simulink model "mcb_pmsm_hall_offset_MCSPTE1AK144"  (R2021a)
settings: Solver=FixedStepDiscrete  StartTime=0.0  StopTime=10.0  FixedStep=0.001  RelTol=1e-3  EnableMultiTasking=on
PreLoadFcn:
  | mcb_pmsm_foc_hall_MCSPTE1AK144_data;
InitFcn:
  | mbd_s32k_consistency_checks(bdroot(gcs));
values from neighbouring files (symbols this model uses):
  PWM_frequency = 20e3    (= 20000)    [mcb_pmsm_foc_hall_MCSPTE1AK144_data.m]
  Ts = T_pwm * 2    (= 0.0001)    [mcb_pmsm_foc_hall_MCSPTE1AK144_data.m]
  Ts_uart = 0.01    [mcb_pmsm_foc_hall_MCSPTE1AK144_data.m]
undefined symbols (not defined in the file or in its folder): External, LQFP, One, pmsm, Shot, TRGMUX_PDB_TRIG
libraries: mbd_s32k1xx_ec_toolbox x34, simulink x9, mcbcontrolslib x5, hdlsllib x4, mbd_msd_ec_toolbox x4, mcbpositiondecoderlib x2
settings Model: Creator=nxf40284  LastModifiedBy=Prasad Hegde
settings SolverCC: AlgebraicLoopSolver=TrustRegion
settings DataIOCC: ExternalInput=off  InitialState=off  LimitDataPoints=on  SaveFormat=Array  SaveOutput=off  SignalLogging=off  SaveTime=off
settings OptimizationCC: DefaultParameterBehavior=Inlined  UseFloatMulNetSlope=on  DefaultUnderspecifiedDataType=single  UseSpecifiedMinMax=on  EnhancedBackFolding=on  PassReuseOutputArgsAs=Individual arguments  ZeroExternalMemoryAtStartup=off  ZeroInternalMemoryAtStartup=off  NoFixptDivByZeroProtection=on  EfficientFloat2IntCast=on  EfficientTunableParamExpr=on
settings DebuggingCC: MergeDetectMultiDrivingBlocksExec=none  InheritedTsInSrcMsg=none  MultiTaskDSMMsg=none  SingleTaskRateTransMsg=error  ParameterTunabilityLossMsg=error  UnconnectedInputMsg=error  UnconnectedOutputMsg=error  UnconnectedLineMsg=error  AllowSymbolicDim=off  UnknownTsInhSupMsg=error  SFMachineParentedDataDiag=warning  ArithmeticOperatorsInVariantConditions=warning
settings HardwareCC: ProdBitPerPointer=32  ProdBitPerSizeT=32  ProdBitPerPtrDiffT=32  ProdLargestAtomicInteger=Long  ProdLargestAtomicFloat=Double  ProdWordSize=32  ProdHWDeviceType=ARM Compatible->ARM Cortex
settings SFSimCC: MATLABDynamicMemAlloc=off
settings RTWCC: Description=Model Based Design Toolbox S32K1xx Code Generation Target  SystemTargetFile=mbd_s32k.tlc  MakeCommand=mbd_s32k_make_rtw COPY_MDLREF_INCLUDES=0  TemplateMakefile=mbd_s32k.tmf
settings CodeAppCC: ForceParamTrailComments=on  IgnoreCustomStorageClasses=off  OperatorAnnotations=on  SimulinkDataObjDesc=on  SFDataObjDesc=on  InsertBlockDesc=on  StateflowObjectComments=on
settings STFCustomTargetCC: MultiwordLength=256  CombineOutputUpdateFcns=on  ERTCustomFileBanners=on  SupportContinuousTime=off  SupportNonInlinedSFcns=off  MATLABClassNameForMDSCustomization=Simulink.SoftwareTarget.ERTCustomization  GRTInterface=off  UseToolchainInfoCompliant=off  SystemTargetFile=mbd_s32k.tlc
settings ERTTargetCC: ParMdlRefBuildCompliant=off  CompOptLevelCompliant=off  ConcurrentExecutionCompliant=off  RemoveResetFunc=off  ModelStepFunctionPrototypeControlCompliant=off  CPPClassGenCompliant=off  UseToolchainInfoCompliant=off  InlinedParameterPlacement=NonHierarchical  ERTSrcFileBannerTemplate=mbd_ert_code_template.cgt  ERTHdrFileBannerTemplate=mbd_ert_code_template.cgt  ERTDataSrcFileTemplate=mbd_ert_code_template.cgt  ERTDataHdrFileTemplate=mbd_ert_code_template.cgt  ERTCustomFileTemplate=example_file_process.tlc

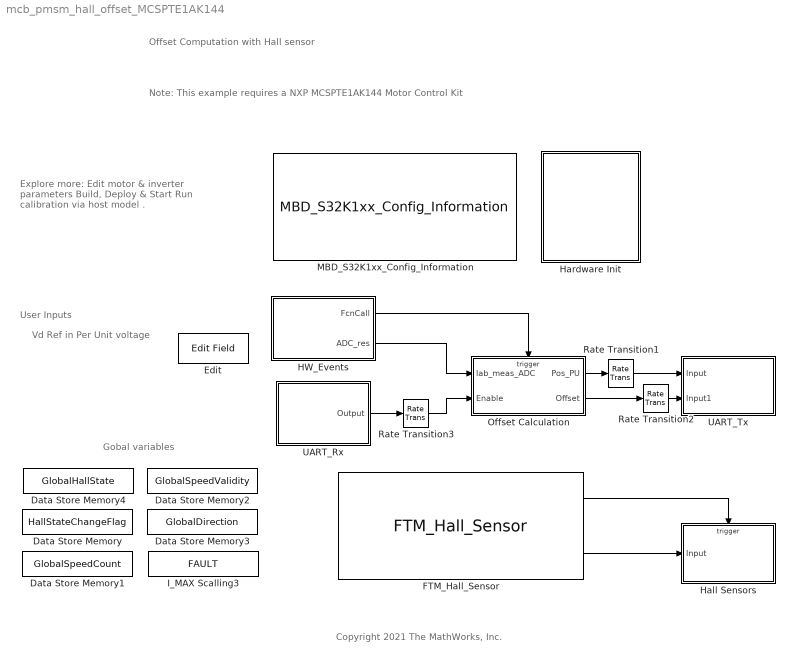
== system mcb_pmsm_hall_offset_MCSPTE1AK144 ==
  note: Note: This example requires a NXP MCSPTE1AK144 Motor Control Kit
  note: User Inputs
  note: Offset Computation with Hall sensor
  note: Vd Ref in Per Unit
      | voltage
  note: Gobal variables
  note: Copyright 2021 The MathWorks, Inc.
  note: Explore more:
      | Edit motor & inverter parameters
      | Build, Deploy & Start
      | Run calibration via host model .
  Data Store Memory : DataStoreMemory  DataStoreName=HallStateChangeFlag  ShowAdditionalParam=off
  Data Store Memory1 : DataStoreMemory  DataStoreName=GlobalSpeedCount  ShowAdditionalParam=off  OutDataTypeStr=uint16
  Data Store Memory2 : DataStoreMemory  DataStoreName=GlobalSpeedValidity  ShowAdditionalParam=off
  Data Store Memory3 : DataStoreMemory  DataStoreName=GlobalDirection  ShowAdditionalParam=off
  Data Store Memory4 : DataStoreMemory  DataStoreName=GlobalHallState  ShowAdditionalParam=off  OutDataTypeStr=uint32
  Edit : EditField  LabelPosition=Hide  ShowInitialText=on  Alignment=Center
  FTM_Hall_Sensor : mbd_s32k1xx_ec_toolbox/Motor Control Blocks/FTM Blocks/FTM_Hall_Sensor  e_mode=Rising or Falling  prescaler=128  max_period=0.10486  isrlevel=5  mcuTargetUpdate=on  filter_en=off  filter_value=0  pinFtm1Ch1=PTA1: [FTM1_CH1 | FTM Channel]  pinFtm2Ch0=PTD10: [FTM2_CH0 | FTM Channel]  pinFtm2Ch1=PTD11: [FTM2_CH1 | FTM Channel]
  HW_Events : Subsystem  TreatAsAtomicUnit=on
  Hall Sensors : Subsystem
  Hardware Init : Subsystem  Priority=2  TreatAsAtomicUnit=on
  I_MAX Scalling3 : DataStoreMemory  DataStoreName=FAULT  ReadBeforeWriteMsg=warning  WriteAfterWriteMsg=warning  WriteAfterReadMsg=warning  ShowAdditionalParam=off  OutDataTypeStr=boolean
  MBD_S32K1xx_Config_Information : mbd_s32k1xx_ec_toolbox/MBD_S32K1xx_Config_Information  Priority=1  mbdt_ver=0  disp_str=|  config_params=[]  mcu_target_name=S32K144  mcu_target_package=100-LQFP  mcu_target_sram_size=64KB  mcu_system_clock_freq=80  mcu_xtal_freq=External 8  mcu_steptick_timer=LPIT Channel 0  mcu_steptick_prio=10  ds_import_enable=on  target_compiler=GCC  target_memory=FLASH  gcc_target_compile_opts=-mcpu=cortex-m4 -mthumb -mfloat-abi=hard -mfpu=fpv4-sp-d16 -O1 -g -gstrict-dwarf  gcc_target_assemble_opts=-mcpu=cortex-m4 -mthumb -mfloat-abi=hard -mfpu=fpv4-sp-d16 -g  gcc_target_link_opts=-mcpu=cortex-m4 -mthumb -mfloat-abi=hard -mfpu=fpv4-sp-d16  gcc_target_default_lcf=on  gcc_target_user_lcf=S32K148_192_flash.ld  ghs_target_compile_opts=-cpu=cortexm4f -thumb -DARM_MATH_CM4 -fpu=vfpv4_d16 -fsingle -Ogeneral -Wundef -Wimplicit-int -Wshadow -Wtrigraphs --no_commons --gnu_asm -gnu99 -gdwarf-2 -G  ghs_target_assemble_opts=-cpu=cortexm4f -fpu=vfpv4_d16  ghs_target_link_opts=-cpu=cortexm4f -thumb -fpu=vfpv4_d16  ghs_target_default_lcf=on  ghs_target_user_lcf=S32K148_192_flash.ld  iar_target_compile_opts=--cpu=Cortex-M4F --thumb --fpu=VFPv4_sp -Ol -e --debug --dlib_config normal  iar_target_assemble_opts=--cpu Cortex-M4F --thumb --fpu VFPv4_sp  iar_target_link_opts=--no_exceptions --vfe --inline  iar_target_default_lcf=on  iar_target_user_lcf=S32K148_192_flash.icf  pil_download_enable=off  rbl_download_enable=on  rbl_start_delay=5000  rbl_download_interface=OpenSDA  rbl_restart_request=off  rbl_com_port=Custom  rbl_com_port_custom=COM1  pil_download_rate=57600  pil_opensda_drive=Custom  pil_opensda_drive_custom=D  pil_uart_instance=1  pil_uart_rx=PTC6: [LPUART1_RX | Receive]  pil_uart_tx=PTC7: [LPUART1_TX | Transmit]  FTM_PWM_PcrCheckEnDis=on  FTM_Input_Edge_Inputs_PcrCheckEnDis=on  FTM_Dual_Edge_Inputs_PcrCheckEnDis=on  FTM_Quadrature_Inputs_PcrCheckEnDis=on  FTM_Hall_Sensor_Inputs_PcrCheckEnDis=on  LPTMR_PcrCheckEnDis=on  PIT_PcrCheckEnDis=on  RTC_PcrCheckEnDis=on  FlexCAN_PcrCheckEnDis=on  LIN_PcrCheckEnDis=on  FlexIO_PcrCheckEnDis=on  LPI2C_PcrCheckEnDis=on  LPSPI_PcrCheckEnDis=on  LPUART_PcrCheckEnDis=on  CMP_PcrCheckEnDis=on  GPIO_OutputPcrCheckEnDis=on  GPIO_InputPcrCheckEnDis=on  SBC_PcrCheckEnDis=on  BMS_PcrCheckEnDis=on  AMMCLIB_PcrCheckEnDis=on  FM_PcrCheckEnDis=on  Profile_PcrCheckEnDis=on  ConfigParams_PcrCheckEnDis=on  ModelRef_PcrCheckEnDis=on  PDB0_PcrCheckEnDis=on  CSEc_PcrCheckEnDis=on  eDMA_PcrCheckEnDis=on  FLASH_PcrCheckEnDis=on  ADC_PcrCheckEnDis=on  WDOG_PcrCheckEnDis=on
      | Target : S32K144-64KB_SRAM
      | Package : 100-pin
      | System clock : 80 MHz
      | XTAL clock : External 8 MHz
      | Compiler : IAR
      | Target Type : FLASH
      | Download Code after build : off
      | Step Tick Interrupt Priority : 15
  Offset Calculation : Subsystem
  Rate Transition1 : RateTransition
  Rate Transition2 : RateTransition
  Rate Transition3 : RateTransition
  UART_Rx : Subsystem
  UART_Tx : Subsystem  TreatAsAtomicUnit=on  SystemSampleTime=Ts_uart
  wires:
  HW_Events/2(ADC_res) -> Offset Calculation/1(Iab_meas_ADC)
  HW_Events/1(FcnCall) -> Offset Calculation/Trigger
  FTM_Hall_Sensor/1 -> Hall Sensors/Trigger
  FTM_Hall_Sensor/2 -> Hall Sensors/1(Input)
  Offset Calculation/2(Offset) -> Rate Transition2/1
  Rate Transition2/1 -> UART_Tx/2(Input1)
  Rate Transition1/1 -> UART_Tx/1(Input)
  Offset Calculation/1(Pos_PU) -> Rate Transition1/1
  UART_Rx/1(Output) -> Rate Transition3/1
  Rate Transition3/1 -> Offset Calculation/2(Enable)

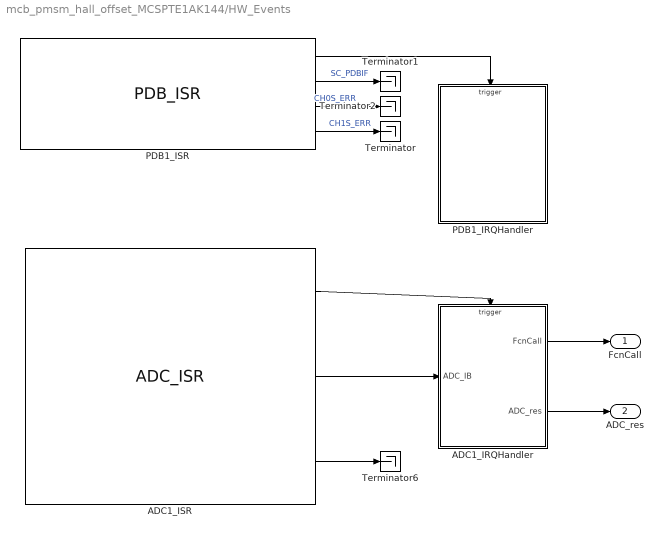
== system mcb_pmsm_hall_offset_MCSPTE1AK144/HW_Events ==
  ADC1_IRQHandler : Subsystem  TreatAsAtomicUnit=on
  ADC1_ISR : mbd_s32k1xx_ec_toolbox/Motor Control Blocks/ADC Blocks/ADC_ISR  instance=1  pri=4  sc1n=A
  PDB1_IRQHandler : Subsystem  TreatAsAtomicUnit=on
  PDB1_ISR : mbd_s32k1xx_ec_toolbox/Motor Control Blocks/PDB Blocks/PDB_ISR  Priority=8  pdbModule=1  prioInterrupt=6  regScPdbie=on  regScPdbeie=off  regIdlyIdly=4999
  Terminator{,1..2,6} (4 alike) : Terminator
  FcnCall : Outport  VectorParamsAs1DForOutWhenUnconnected=off
  ADC_res : Outport  Port=2  VectorParamsAs1DForOutWhenUnconnected=off
  wires:
  ADC1_ISR/3 -> Terminator6/1
  ADC1_IRQHandler/1(FcnCall) -> FcnCall/1
  ADC1_ISR/1 -> ADC1_IRQHandler/Trigger
  PDB1_ISR/3 -> Terminator2/1  "CH0S_ERR"
  PDB1_ISR/4 -> Terminator/1  "CH1S_ERR"
  ADC1_ISR/2 -> ADC1_IRQHandler/1(ADC_IB)
  PDB1_ISR/2 -> Terminator1/1  "SC_PDBIF"
  PDB1_ISR/1 -> PDB1_IRQHandler/Trigger
  ADC1_IRQHandler/2(ADC_res) -> ADC_res/1

== system mcb_pmsm_hall_offset_MCSPTE1AK144/Hall Sensors ==
  Input : Inport
  function : TriggerPort  TriggerType=function-call  VariantControl=Variant
  Halls : Subsystem  Priority=2  TreatAsAtomicUnit=on
      settings: MinAlgLoopOccurrences=on
  wires:
  Input/1 -> Halls/1(Input)  "HallCntEventReg"

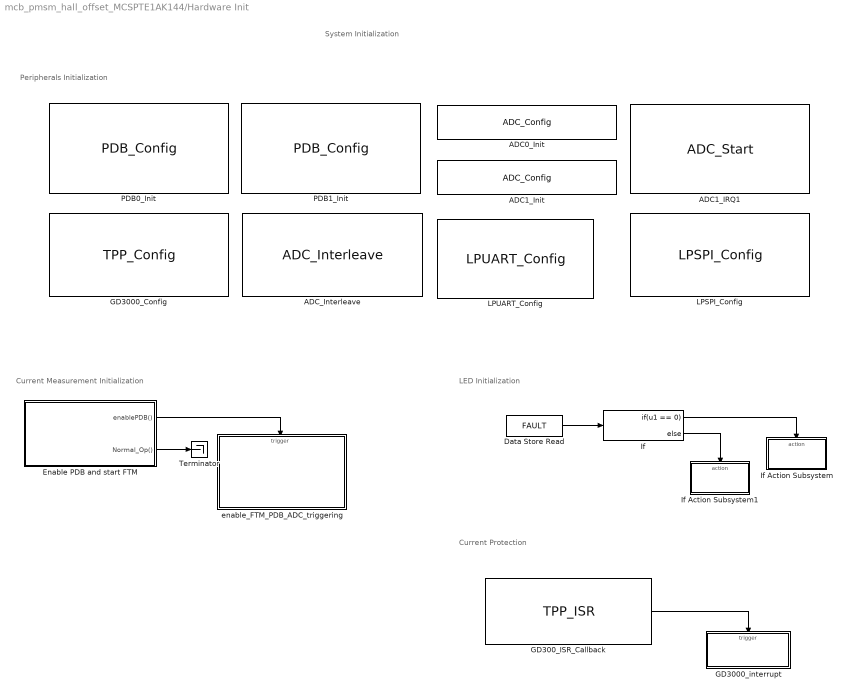
== system mcb_pmsm_hall_offset_MCSPTE1AK144/Hardware Init ==
  note: Current Protection
  note: System Initialization
  note: Peripherals Initialization
  note: Current Measurement Initialization
  note: LED Initialization
  ADC0_Init : mbd_s32k1xx_ec_toolbox/Motor Control Blocks/ADC Blocks/ADC_Config  Priority=3  instance=0  mode=12-bit conversion  smplts=2  adiclk=alternate clock 1  adiv=input clock  show_adv_opts=on  pretrgsel=PDB pre-trigger  swpretrg=Disabled  adtrg=hardware  trgsel=PDB output  refsel=Vrefh and Vrefl  supply_monitoring=off  acfe=off  acfgt=off  acren=off  cv1=0  cv2=0  adco=off  avge=off  avgs=4 samples
  ADC1_IRQ1 : mbd_s32k1xx_ec_toolbox/Motor Control Blocks/ADC Blocks/ADC_Start  Priority=5  instance=1  adc_r=A  adc_chan=PTB16: [ADC1_SE15 | ADC Single Ended Input]  aien=on  mcuTargetUpdate=on
  ADC1_Init : mbd_s32k1xx_ec_toolbox/Motor Control Blocks/ADC Blocks/ADC_Config  Priority=4  instance=1  mode=12-bit conversion  smplts=2  adiclk=alternate clock 1  adiv=input clock  show_adv_opts=on  pretrgsel=PDB pre-trigger  swpretrg=Disabled  adtrg=hardware  trgsel=PDB output  refsel=Vrefh and Vrefl  supply_monitoring=off  acfe=off  acfgt=off  acren=off  cv1=0  cv2=0  adco=off  avge=off  avgs=4 samples
  ADC_Interleave : mbd_s32k1xx_ec_toolbox/Motor Control Blocks/ADC Blocks/ADC_Interleave  adcInterleavePins=PTB1 to ADC0_SE5 and ADC1_SE15  adcInterleaveInit=on
  Data Store Read : DataStoreRead  DataStoreName=FAULT  IndexOptions=Index vector (dialog)  Indices=1  OutputSizes=1
  Enable PDB and start FTM : Stateflow chart  TreatAsAtomicUnit=on
  GD3000_Config : mbd_msd_ec_toolbox/TPP/TPP_Config  Priority=1  tppInstance=0  desatMode=on  fullonMode=off  lockMode=off  overtempEvent=on  phaseEvent=off  desatEvent=off  framingEvent=on  vlsEvent=on  writeErrEvent=on  overcurrentEvent=on  resetEvent=on  mcuTppIntEn=off  prioInt=15  tppDeadtime=500  initTppNow=on  tppSpiInst=Please add SPI block to workspace  tppPwmModule=Please add FTM block to workspace  tppPair0_1=on  tppPair2_3=on  tppPair4_5=on  tppPair6_7=off  tppFirstChHS=on  tppEn1Pin=PTA2: [PTA2 | Port A I/O]  tppEn2Pin=PTA2: [PTA2 | Port A I/O]  tppRstPin=PTA3: [PTA3 | Port A I/O]  tppCsPin=PTB5: [PTB5 | Port B I/O]  tppIntPin=PTE10: [PTE10 | Port E I/O]
  GD3000_interrupt : Subsystem  TreatAsAtomicUnit=on
  "GD300_ISR_Callback " : mbd_msd_ec_toolbox/TPP/TPP_ISR  tppInstance=0
  If : If  IfExpression=u1 == 0
  If Action Subsystem : Subsystem  TreatAsAtomicUnit=on
  If Action Subsystem1 : Subsystem  TreatAsAtomicUnit=on
  "LPSPI_Config " : mbd_s32k1xx_ec_toolbox/Communication Blocks/SPI Blocks/LPSPI_Config   InstanceNumber=0  Role=Master  BaudRate=1000000  ShowAdvanced=on  sin=PTB3: [LPSPI0_SIN | LPSPI Serial Data Input]  sout=PTB4: [LPSPI0_SOUT | LPSPI Serial Data Output]  sck=PTB2: [LPSPI0_SCK | LPSPI Serial Clock I/O]  pcs0=None  pcs1=PTB5: [LPSPI0_PCS1 | Peripheral Chip Select 1]  pcs2=None  pcs3=None  CPHA=1  CPOL=0  BitOrder=MSB first  TransferSize=8  WhichPCS=1  PCSPol=ActiveLow  ContinuousTransfer=off
  LPUART_Config : mbd_s32k1xx_ec_toolbox/Communication Blocks/UART Blocks/LPUART_Config  Priority=1  instance=1  baudrate=256000  databits=8  parity=None  sbns=1  bothedge=rising edge  rxinv=off  txinv=off  show_adv_opts=on  brk13=13 - 16 bit times  lbkde=13 - 16 bit times  rx=PTC6: [LPUART1_RX | Receive]  tx=PTC7: [LPUART1_TX | Transmit]  cts=PTA6: [LPUART1_CTS | Clear To Send (bar)]  rts=PTA7: [LPUART1_RTS | Request To Send]
  PDB0_Init : mbd_s32k1xx_ec_toolbox/Motor Control Blocks/PDB Blocks/PDB_Config  Priority=1  pdbModule=0  regScCont=One-Shot  regScTrgsel=External (TRGMUX_PDB_TRIG)  trgMuxSel=FTM3 Initialize Trigger  trgMuxSelPin=PTB5: [TRGMUX_IN0 | Trigger Mux Input]  regModModulus=5000  regScPrescaler=1  regScMult=1  regPoenPoen0=off  regPo0DlyDly1=0  regPo0DlyDly2=0  enable_pdb_init=off  show_adv_opts=on  regCh0C1En0=on  regCh0C1En1=off  regCh0C1En2=off  regCh0C1En3=off  regCh0C1En4=off  regCh0C1En5=off  regCh0C1En6=off  regCh0C1En7=off  regCh0C1Bb0=off  regCh0C1Bb1=off  regCh0C1Bb2=off  regCh0C1Bb3=off  regCh0C1Bb4=off  regCh0C1Bb5=off  regCh0C1Bb6=off  regCh0C1Bb7=off  regCh0C1Tos0=Pre-trigger is in delay mode  regCh0C1Tos1=Pre-trigger is in delay mode  regCh0C1Tos2=Pre-trigger is in delay mode  regCh0C1Tos3=Pre-trigger is in delay mode  regCh0C1Tos4=Pre-trigger is in delay mode  regCh0C1Tos5=Pre-trigger is in delay mode  regCh0C1Tos6=Pre-trigger is in delay mode  regCh0C1Tos7=Pre-trigger is in delay mode  regCh0DlyDly0=2000  regCh0DlyDly1=0  regCh0DlyDly2=0  regCh0DlyDly3=0  regCh0DlyDly4=0  regCh0DlyDly5=0  regCh0DlyDly6=0  regCh0DlyDly7=0  regCh1C1En0=off  regCh1C1En1=off  regCh1C1En2=off  regCh1C1En3=off  regCh1C1En4=off  regCh1C1En5=off  regCh1C1En6=off  regCh1C1En7=off  regCh1C1Bb0=off  regCh1C1Bb1=off  regCh1C1Bb2=off  regCh1C1Bb3=off  regCh1C1Bb4=off  regCh1C1Bb5=off  regCh1C1Bb6=off  regCh1C1Bb7=off  regCh1C1Tos0=Pre-trigger is in delay mode  regCh1C1Tos1=Pre-trigger is in delay mode  regCh1C1Tos2=Pre-trigger is in delay mode  regCh1C1Tos3=Pre-trigger is in delay mode  regCh1C1Tos4=Pre-trigger is in delay mode  regCh1C1Tos5=Pre-trigger is in delay mode  regCh1C1Tos6=Pre-trigger is in delay mode  regCh1C1Tos7=Pre-trigger is in delay mode  regCh1DlyDly0=0  regCh1DlyDly1=0  regCh1DlyDly2=0  regCh1DlyDly3=0  regCh1DlyDly4=0  regCh1DlyDly5=0  regCh1DlyDly6=0  regCh1DlyDly7=0
  PDB1_Init : mbd_s32k1xx_ec_toolbox/Motor Control Blocks/PDB Blocks/PDB_Config  Priority=2  pdbModule=1  regScCont=One-Shot  regScTrgsel=External (TRGMUX_PDB_TRIG)  trgMuxSel=FTM3 Initialize Trigger  trgMuxSelPin=PTB5: [TRGMUX_IN0 | Trigger Mux Input]  regModModulus=5000  regScPrescaler=1  regScMult=1  regPoenPoen0=off  regPo0DlyDly1=0  regPo0DlyDly2=0  enable_pdb_init=off  show_adv_opts=on  regCh0C1En0=on  regCh0C1En1=off  regCh0C1En2=off  regCh0C1En3=off  regCh0C1En4=off  regCh0C1En5=off  regCh0C1En6=off  regCh0C1En7=off  regCh0C1Bb0=off  regCh0C1Bb1=off  regCh0C1Bb2=off  regCh0C1Bb3=off  regCh0C1Bb4=off  regCh0C1Bb5=off  regCh0C1Bb6=off  regCh0C1Bb7=off  regCh0C1Tos0=Pre-trigger is in delay mode  regCh0C1Tos1=Pre-trigger is in delay mode  regCh0C1Tos2=Pre-trigger is in delay mode  regCh0C1Tos3=Pre-trigger is in delay mode  regCh0C1Tos4=Pre-trigger is in delay mode  regCh0C1Tos5=Pre-trigger is in delay mode  regCh0C1Tos6=Pre-trigger is in delay mode  regCh0C1Tos7=Pre-trigger is in delay mode  regCh0DlyDly0=2000  regCh0DlyDly1=0  regCh0DlyDly2=0  regCh0DlyDly3=0  regCh0DlyDly4=0  regCh0DlyDly5=0  regCh0DlyDly6=0  regCh0DlyDly7=0  regCh1C1En0=off  regCh1C1En1=off  regCh1C1En2=off  regCh1C1En3=off  regCh1C1En4=off  regCh1C1En5=off  regCh1C1En6=off  regCh1C1En7=off  regCh1C1Bb0=off  regCh1C1Bb1=off  regCh1C1Bb2=off  regCh1C1Bb3=off  regCh1C1Bb4=off  regCh1C1Bb5=off  regCh1C1Bb6=off  regCh1C1Bb7=off  regCh1C1Tos0=Pre-trigger is in delay mode  regCh1C1Tos1=Pre-trigger is in delay mode  regCh1C1Tos2=Pre-trigger is in delay mode  regCh1C1Tos3=Pre-trigger is in delay mode  regCh1C1Tos4=Pre-trigger is in delay mode  regCh1C1Tos5=Pre-trigger is in delay mode  regCh1C1Tos6=Pre-trigger is in delay mode  regCh1C1Tos7=Pre-trigger is in delay mode  regCh1DlyDly0=0  regCh1DlyDly1=0  regCh1DlyDly2=0  regCh1DlyDly3=0  regCh1DlyDly4=0  regCh1DlyDly5=0  regCh1DlyDly6=0  regCh1DlyDly7=0
  Terminator : Terminator
  enable_FTM_PDB_ADC_triggering : Subsystem  TreatAsAtomicUnit=on
      settings: RTWSystemCode=Inline
  wires:
  Enable PDB and start FTM/1(enablePDB()) -> enable_FTM_PDB_ADC_triggering/Trigger
  Enable PDB and start FTM/2(Normal_Op()) -> Terminator/1
  If/1 -> If Action Subsystem/Action
  Data Store Read/1 -> If/1
  "GD300_ISR_Callback "/1 -> GD3000_interrupt/Trigger
  If/2 -> If Action Subsystem1/Action

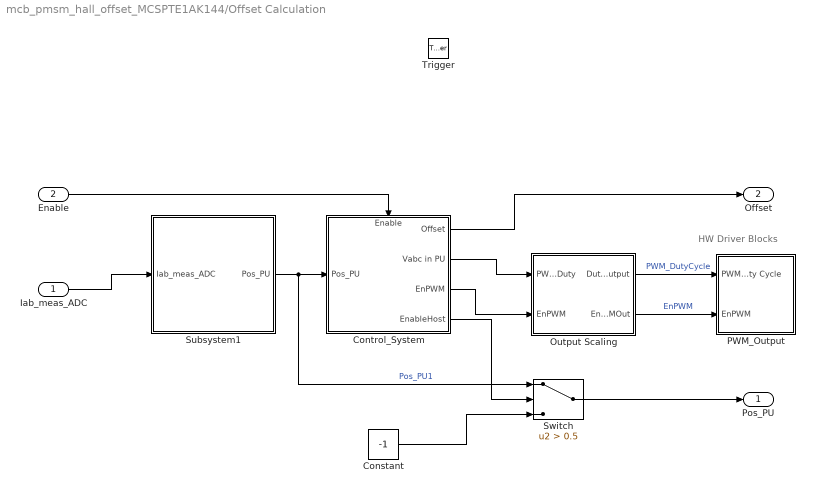
== system mcb_pmsm_hall_offset_MCSPTE1AK144/Offset Calculation ==
  note: HW Driver Blocks
  Iab_meas_ADC : Inport
  Enable : Inport  Port=2
  Trigger : TriggerPort  TriggerType=function-call  VariantControl=Variant
  Constant : Constant  Value=-1  OutDataTypeStr=dataType
  Control_System : Subsystem  Priority=2  TreatAsAtomicUnit=on
      settings: PortSchema="{\"entries\":[{\"content\":{\"sides\":[{\"content\":{\"connectorIds\":[\"In1\"]},\"type\":\"ConnectorPlacement.EquallySpacedRectSide\",\"uuid\":\"173f19dc-215a-42db-973a-f41a5d08ea9f\"},{\"content\":{\"connectorIds\":[\"Out1\",\"Out2\",\"Out3\",\"Out4\"],\"side\":\"RIGHT\"},\"type\":\"ConnectorPlacement.EquallySpacedRectSide\",\"uuid\":\"cd99c6ca-9263-4750-8ed8-89a3541b6698\"},{\"content\":{\"connectorIds\":[\"In2\"],\"side\":\"TOP\"},\"type\":\"ConnectorPlacement.EquallySpacedRectSide\",\"uuid\":\"772cacff-5f94-49f6-b032-a432d84880d4\"}]},\"type\":\"ConnectorPlacement.EquallySpacedConnector\",\"uuid\":\"848ecd11-ed94-43c1-b606-fea732c678b8\"}],\"packageUris\":[\"http://schema.mathworks.com/mf0/Connector/R2020b\"],\"version\":\"1.0\"}"
  Output Scaling : Subsystem  Priority=3  TreatAsAtomicUnit=on
  PWM_Output : Subsystem  Priority=4  TreatAsAtomicUnit=on
  Subsystem1 : Subsystem  Priority=1  TreatAsAtomicUnit=on
      settings: MinAlgLoopOccurrences=on
  Switch : Switch  Criteria=u2 > Threshold  Threshold=0.5
  Pos_PU : Outport
  Offset : Outport  Port=2
  wires:
  Switch/1 -> Pos_PU/1
  Control_System/1(Offset) -> Offset/1
  Enable/1 -> Control_System/2(Enable)
  Constant/1 -> Switch/3
  Control_System/4(EnableHost) -> Switch/2
  Control_System/2(Vabc in PU) -> Output Scaling/1(PWM_Duty)
  Output Scaling/1(Duty Output) -> PWM_Output/1(PWM_Duty Cycle)  "PWM_DutyCycle"
  Iab_meas_ADC/1 -> Subsystem1/1(Iab_meas_ADC)
  Control_System/3(EnPWM) -> Output Scaling/2(EnPWM)
  Subsystem1/1(Pos_PU) -> Switch/1, Control_System/1(Pos_PU)  "Pos_PU1"
  Output Scaling/2(EnPWMOut) -> PWM_Output/2(EnPWM)  "EnPWM"

== system mcb_pmsm_hall_offset_MCSPTE1AK144/UART_Rx ==
  Constant : Constant  OutDataTypeStr=Inherit: Inherit via back propagation
  Data Type Conversion2 : DataTypeConversion  RndMeth=Simplest
  LPUART_Receive : mbd_s32k1xx_ec_toolbox/Communication Blocks/UART Blocks/LPUART_Receive  instance=1
  Output : Outport
  wires:
  Constant/1 -> LPUART_Receive/1
  LPUART_Receive/1 -> Data Type Conversion2/1
  Data Type Conversion2/1 -> Output/1

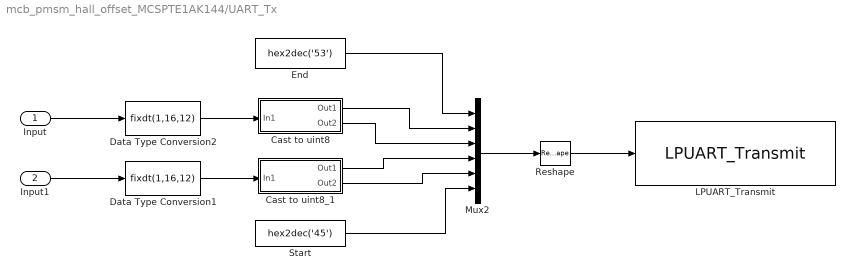
== system mcb_pmsm_hall_offset_MCSPTE1AK144/UART_Tx ==
  Input : Inport
  Input1 : Inport  Port=2
  Cast to uint8 : Subsystem
  Cast to uint8_1 : Subsystem
  Data Type Conversion1 : DataTypeConversion  OutDataTypeStr=fixdt(1,16,12)  RndMeth=Simplest
  Data Type Conversion2 : DataTypeConversion  OutDataTypeStr=fixdt(1,16,12)  RndMeth=Simplest
  End : Constant  Value=hex2dec('53')  OutDataTypeStr=uint8
  LPUART_Transmit : mbd_s32k1xx_ec_toolbox/Communication Blocks/UART Blocks/LPUART_Transmit  Priority=2  instance=1
  Mux2 : Mux  Inputs=6
  Reshape : Reshape
  Start : Constant  Value=hex2dec('45')  OutDataTypeStr=uint8
  wires:
  Start/1 -> Mux2/6
  End/1 -> Mux2/1
  Reshape/1 -> LPUART_Transmit/1
  Mux2/1 -> Reshape/1
  Input1/1 -> Data Type Conversion1/1
  Input/1 -> Data Type Conversion2/1
  Data Type Conversion1/1 -> Cast to uint8_1/1(In1)
  Cast to uint8/1(Out1) -> Mux2/2
  Cast to uint8/2(Out2) -> Mux2/3
  Cast to uint8_1/1(Out1) -> Mux2/4
  Cast to uint8_1/2(Out2) -> Mux2/5
  Data Type Conversion2/1 -> Cast to uint8/1(In1)

== system mcb_pmsm_hall_offset_MCSPTE1AK144/HW_Events/ADC1_IRQHandler ==
  ADC_IB : Inport
  function : TriggerPort  TriggerType=function-call  VariantControl=(inherit)
  ADC_AD4_IA : mbd_s32k1xx_ec_toolbox/Motor Control Blocks/ADC Blocks/ADC_Start  Priority=2  instance=0  adc_r=A  adc_chan=PTB0: [ADC0_SE4 | ADC Single Ended Input]  aien=off  mcuTargetUpdate=on
  FTM_Init_Trigger_Disable : mbd_s32k1xx_ec_toolbox/Motor Control Blocks/FTM Blocks/FTM_Init_Trigger_Disable_Enable  Priority=1  ftmModule=3  action=Disable
  Function-Call Generator : simulink/Ports & Subsystems/Function-Call Generator  sample_time=-1  numberOfIterations=1  DisallowWideOutput=off
  Mux : Mux  Inputs=2
  FcnCall : Outport  VectorParamsAs1DForOutWhenUnconnected=off
  ADC_res : Outport  Port=2  VectorParamsAs1DForOutWhenUnconnected=off
  wires:
  ADC_AD4_IA/1 -> Mux/1  "ADC_IA"
  Mux/1 -> ADC_res/1
  Function-Call Generator/1 -> FcnCall/1
  ADC_IB/1 -> Mux/2  "ADC_IB"

== system mcb_pmsm_hall_offset_MCSPTE1AK144/HW_Events/PDB1_IRQHandler ==
  function : TriggerPort  TriggerType=function-call  VariantControl=(inherit)
  FTM_Init_Trigger_Enable : mbd_s32k1xx_ec_toolbox/Motor Control Blocks/FTM Blocks/FTM_Init_Trigger_Disable_Enable  ftmModule=3  action=Enable

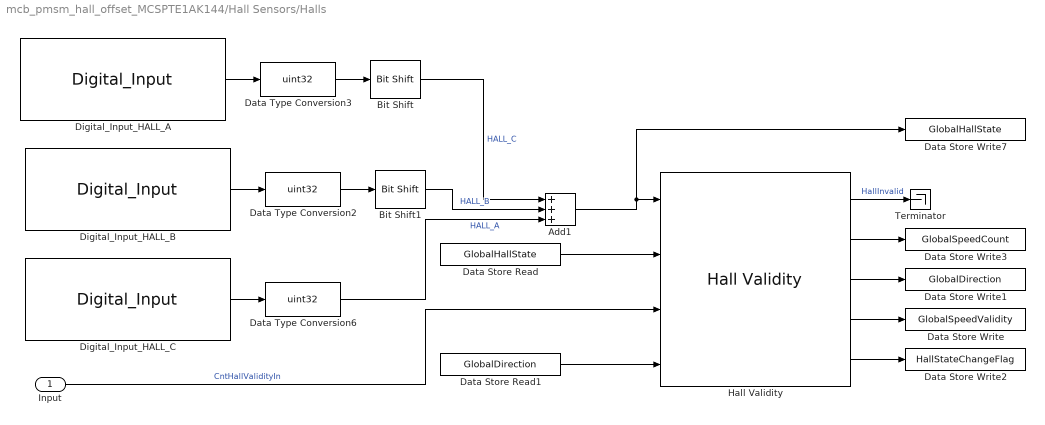
== system mcb_pmsm_hall_offset_MCSPTE1AK144/Hall Sensors/Halls ==
  Input : Inport
  Add1 : Sum  Inputs=+++  OutDataTypeStr=Inherit: Inherit via back propagation
  Bit Shift : hdlsllib/Logic and Bit Operations/Bit Shift  mode=Shift Left Logical  N=2
  Bit Shift1 : hdlsllib/Logic and Bit Operations/Bit Shift  mode=Shift Left Logical  N=1
  Data Store Read : DataStoreRead  DataStoreName=GlobalHallState  IndexOptions=Index vector (dialog)  Indices=1  OutputSizes=1
  Data Store Read1 : DataStoreRead  DataStoreName=GlobalDirection  IndexOptions=Index vector (dialog)  Indices=1  OutputSizes=1
  Data Store Write : DataStoreWrite  DataStoreName=GlobalSpeedValidity  IndexOptions=Index vector (dialog)  Indices=1  OutputSizes=1
  Data Store Write1 : DataStoreWrite  DataStoreName=GlobalDirection  IndexOptions=Index vector (dialog)  Indices=1  OutputSizes=1
  Data Store Write2 : DataStoreWrite  DataStoreName=HallStateChangeFlag  IndexOptions=Index vector (dialog)  Indices=1  OutputSizes=1
  Data Store Write3 : DataStoreWrite  DataStoreName=GlobalSpeedCount  IndexOptions=Index vector (dialog)  Indices=1  OutputSizes=1
  Data Store Write7 : DataStoreWrite  Priority=1  DataStoreName=GlobalHallState  IndexOptions=Index vector (dialog)  Indices=1  OutputSizes=1
  Data Type Conversion2 : DataTypeConversion  OutDataTypeStr=uint32
  Data Type Conversion3 : DataTypeConversion  OutDataTypeStr=uint32
  Data Type Conversion6 : DataTypeConversion  OutDataTypeStr=uint32
  Digital_Input_HALL_A : mbd_s32k1xx_ec_toolbox/GPIO Blocks/Digital_Input  gpio_pin=PTA1: [PTA1 | Port A I/O]  pull_resistor=None  passive_filter=off
  Digital_Input_HALL_B : mbd_s32k1xx_ec_toolbox/GPIO Blocks/Digital_Input  gpio_pin=PTD10: [PTD10 | Port D I/O]  pull_resistor=None  passive_filter=off
  Digital_Input_HALL_C : mbd_s32k1xx_ec_toolbox/GPIO Blocks/Digital_Input  gpio_pin=PTD11: [PTD11 | Port D I/O]  pull_resistor=None  passive_filter=off
  Hall Validity : mcbpositiondecoderlib/Hall Validity  hallSequence=ABC  sequence=[5,4,6,2,3,1]  CounterSize=16 bits
      settings: SourceProductBaseCode=MT
  Terminator : Terminator
  wires:
  Hall Validity/3 -> Data Store Write1/1
  Hall Validity/4 -> Data Store Write/1
  Hall Validity/5 -> Data Store Write2/1
  Hall Validity/1 -> Terminator/1  "HallInvalid"
  Hall Validity/2 -> Data Store Write3/1
  Data Store Read/1 -> Hall Validity/2
  Data Store Read1/1 -> Hall Validity/4
  Digital_Input_HALL_A/1 -> Data Type Conversion3/1
  Data Type Conversion3/1 -> Bit Shift/1
  Digital_Input_HALL_C/1 -> Data Type Conversion6/1
  Bit Shift1/1 -> Add1/2  "HALL_B"
  Data Type Conversion2/1 -> Bit Shift1/1
  Data Type Conversion6/1 -> Add1/3  "HALL_A"
  Bit Shift/1 -> Add1/1  "HALL_C"
  Digital_Input_HALL_B/1 -> Data Type Conversion2/1
  Add1/1 -> Data Store Write7/1, Hall Validity/1
  Input/1 -> Hall Validity/3  "CntHallValidityIn"

== system mcb_pmsm_hall_offset_MCSPTE1AK144/Hardware Init/GD3000_interrupt ==
  function : TriggerPort  TriggerType=function-call  VariantControl=Variant
  FAULT_write : DataStoreWrite  DataStoreName=FAULT  IndexOptions=Index vector (dialog)  Indices=1  OutputSizes=1
  FTM_PWM_Disable_Enable : mbd_s32k1xx_ec_toolbox/Motor Control Blocks/FTM Blocks/FTM_PWM_Disable_Enable  ftmModule=3  action=Disable
  NOK : Constant  OutDataTypeStr=boolean
  TPP_Functional_Mode : mbd_msd_ec_toolbox/TPP/TPP_Functional_Mode  tppInstance=0  action=Sleep
  wires:
  NOK/1 -> FAULT_write/1

== system mcb_pmsm_hall_offset_MCSPTE1AK144/Hardware Init/If Action Subsystem ==
  Action Port : ActionPort  ActionPortLabel=if(u1 == 0)
  LED_GREEN : Constant  Value=0  OutDataTypeStr=boolean  SampleTime=-1
  LED_GREEN_ON : mbd_s32k1xx_ec_toolbox/GPIO Blocks/Digital_Output  gpio_pin=PTD16: [PTD16 | Port D I/O]  init_val=Low  drive_strength=Low
  LED_RED : Constant  OutDataTypeStr=boolean  SampleTime=-1
  LED_RED_OFF : mbd_s32k1xx_ec_toolbox/GPIO Blocks/Digital_Output  gpio_pin=PTD15: [PTD15 | Port D I/O]  init_val=Low  drive_strength=Low
  wires:
  LED_GREEN/1 -> LED_GREEN_ON/1
  LED_RED/1 -> LED_RED_OFF/1

== system mcb_pmsm_hall_offset_MCSPTE1AK144/Hardware Init/If Action Subsystem1 ==
  Action Port : ActionPort  ActionPortLabel=else
  LED_GREEN_ON : mbd_s32k1xx_ec_toolbox/GPIO Blocks/Digital_Output  gpio_pin=PTD16: [PTD16 | Port D I/O]  init_val=Low  drive_strength=Low
  LED_GREEN_on : Constant  OutDataTypeStr=boolean  SampleTime=-1
  LED_RED_OFF : mbd_s32k1xx_ec_toolbox/GPIO Blocks/Digital_Output  gpio_pin=PTD15: [PTD15 | Port D I/O]  init_val=Low  drive_strength=Low
  LED_RED_off : Constant  Value=0  OutDataTypeStr=boolean  SampleTime=-1
  wires:
  LED_GREEN_on/1 -> LED_GREEN_ON/1
  LED_RED_off/1 -> LED_RED_OFF/1

== system mcb_pmsm_hall_offset_MCSPTE1AK144/Hardware Init/enable_FTM_PDB_ADC_triggering ==
  function : TriggerPort  TriggerType=function-call  VariantControl=(inherit)
  Custom code to reload the PDB value1 : Subsystem  Priority=6  mask(System Outputs){ShowInLibBrowser=0}
      mask prompts: ShowInLibBrowser "Simulink:masks:CustCodeMaskParam1_MP"
      settings: CopyFcn=cccopyfcn(gcb)  OpenFcn=ccopenfcn('System Outputs Function')
      mask Help: eval('feval(''rtwprivate'',''rtwhelpview'',''rtw_sys_outputs_block'')');
      mask Display: disp('System\nOutputs');
  FTM_Init_Trigger_Disable_Enable1 : mbd_s32k1xx_ec_toolbox/Motor Control Blocks/FTM Blocks/FTM_Init_Trigger_Disable_Enable  Priority=3  ftmModule=3  action=Enable
  FTM_PWM_Disable_Enable : mbd_s32k1xx_ec_toolbox/Motor Control Blocks/FTM Blocks/FTM_PWM_Disable_Enable  Priority=1  ftmModule=3  action=Enable
  PDB0_Enable : mbd_s32k1xx_ec_toolbox/Motor Control Blocks/PDB Blocks/PDB_Enable  Priority=4  pdbModule=0  pdbAction=Enable
  PDB1_Enable1 : mbd_s32k1xx_ec_toolbox/Motor Control Blocks/PDB Blocks/PDB_Enable  Priority=5  pdbModule=1  pdbAction=Enable
  "TPP_ISR_Enable_Disable " : mbd_msd_ec_toolbox/TPP/TPP_ISR_Enable_Disable  Priority=4  tppInstance=0  mcuTppIntEn=on  prioInt=13

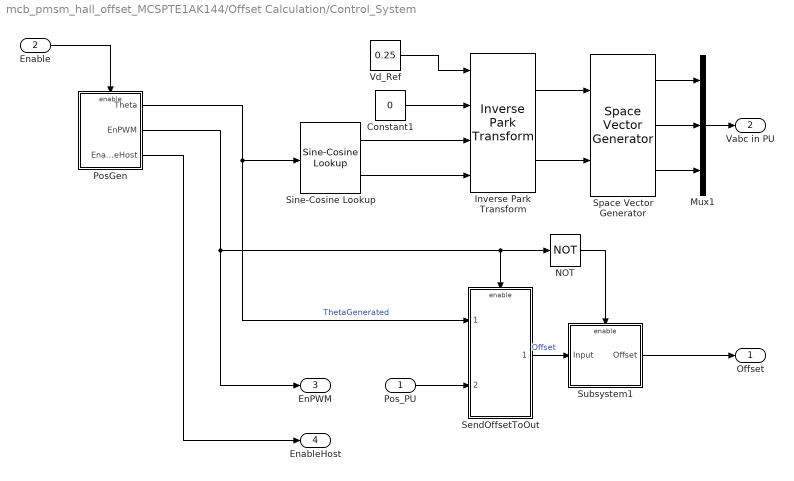
== system mcb_pmsm_hall_offset_MCSPTE1AK144/Offset Calculation/Control_System ==
  Pos_PU : Inport
  Enable : Inport  Port=2
  Constant1 : Constant  Value=0  OutDataTypeStr=dataType  SampleTime=-1
  Inverse Park Transform : mcbcontrolslib/Inverse Park Transform  AxisAlignment=D-axis
  Mux1 : Mux  Inputs=3
  NOT : Logic  Operator=NOT  IconShape=distinctive  AllPortsSameDT=off  OutDataTypeStr=boolean
  PosGen : Subsystem
  SendOffsetToOut : Subsystem
  Sine-Cosine Lookup : mcbcontrolslib/Sine-Cosine Lookup  AngleInput=Per-unit  N_points=1024
      settings: SourceProductBaseCode=MT
  Space Vector Generator : mcbcontrolslib/Space Vector Generator
      settings: SourceProductBaseCode=MT
  Subsystem1 : Subsystem
  Vd_Ref : Constant  Value=0.25  OutDataTypeStr=dataType
  Offset : Outport  VectorParamsAs1DForOutWhenUnconnected=off
  Vabc in PU : Outport  Port=2  VectorParamsAs1DForOutWhenUnconnected=off
  EnPWM : Outport  Port=3  VectorParamsAs1DForOutWhenUnconnected=off
  EnableHost : Outport  Port=4  VectorParamsAs1DForOutWhenUnconnected=off
  wires:
  Inverse Park Transform/1 -> Space Vector Generator/1
  Inverse Park Transform/2 -> Space Vector Generator/2
  Pos_PU/1 -> SendOffsetToOut/2(Theta_hall)
  Space Vector Generator/1 -> Mux1/1
  Space Vector Generator/2 -> Mux1/2
  Space Vector Generator/3 -> Mux1/3
  Mux1/1 -> Vabc in PU/1
  Vd_Ref/1 -> Inverse Park Transform/1
  Constant1/1 -> Inverse Park Transform/2
  PosGen/1(Theta) -> SendOffsetToOut/1(Theta_Open), Sine-Cosine Lookup/1  "ThetaGenerated"
  Sine-Cosine Lookup/1 -> Inverse Park Transform/3
  Sine-Cosine Lookup/2 -> Inverse Park Transform/4
  SendOffsetToOut/1(Offset) -> Subsystem1/1(Input)  "Offset"
  Enable/1 -> PosGen/Enable
  PosGen/2(EnPWM) -> EnPWM/1, SendOffsetToOut/Enable, NOT/1
  NOT/1 -> Subsystem1/Enable
  Subsystem1/1(Offset) -> Offset/1
  PosGen/3(EnableHost) -> EnableHost/1

== system mcb_pmsm_hall_offset_MCSPTE1AK144/Offset Calculation/Output Scaling ==
  PWM_Duty : Inport
  EnPWM : Inport  Port=2
  Constant : Constant  OutDataTypeStr=dataType
  Gain : Gain  Gain=0.5  RndMeth=Simplest  OutDataTypeStr=Inherit: Same as input
  Sum : Sum  Inputs=|++  RndMeth=Simplest  OutDataTypeStr=Inherit: Same as first input
  Duty Output : Outport
  EnPWMOut : Outport  Port=2  VectorParamsAs1DForOutWhenUnconnected=off
  wires:
  PWM_Duty/1 -> Sum/1
  Gain/1 -> Duty Output/1
  Sum/1 -> Gain/1
  Constant/1 -> Sum/2
  EnPWM/1 -> EnPWMOut/1

== system mcb_pmsm_hall_offset_MCSPTE1AK144/Offset Calculation/PWM_Output ==
  PWM_Duty Cycle : Inport
  EnPWM : Inport  Port=2
  Demux1 : Demux  Outputs=3
  FTM_PWM_Config : mbd_s32k1xx_ec_toolbox/Motor Control Blocks/FTM Blocks/FTM_PWM_Config  ftmModule=3  ftmMode=Center-Aligned PWM  ftmSourceClock=80 MHz  swcontrol_enable=off  chan0En=on  chan0Type=Complementary  chan2En=on  chan2Type=Complementary  chan4En=on  chan4Type=Complementary  chan6En=off  chan6Type=Independent  ftmPwmUnits=Hz  outFrequency=20000  ftmPeriod=4000  ftmPrescaler=Divide by 1  deadtimeUnits=Nanoseconds  deadtimeNs=0  deadtimeTicks=0  deadtimePrescaler=Divide by 1  dutyCycleCh0=0  dutyCycleCh1=0  dutyCycleCh2=0  dutyCycleCh3=0  dutyCycleCh4=0  dutyCycleCh5=0  dutyCycleCh6=0.25  dutyCycleCh7=0.25  dutyCycleSim=off  startAfterInit=off  showAdvOpt=on  pinFtmCh0=PTB8: [FTM3_CH0 | FTM Channel]  pinFtmCh1=PTB9: [FTM3_CH1 | FTM Channel]  pinPolCh0=Active Low  pinPolCh1=Active High  outputComplem0=Main duplicated  outputLevel0=High  outputLevel1=Low  pinFtmCh2=PTB10: [FTM3_CH2 | FTM Channel]  pinFtmCh3=PTB11: [FTM3_CH3 | FTM Channel]  pinPolCh2=Active Low  pinPolCh3=Active High  outputComplem2=Main duplicated  outputLevel2=High  outputLevel3=Low  pinFtmCh4=PTC10: [FTM3_CH4 | FTM Channel]  pinFtmCh5=PTC11: [FTM3_CH5 | FTM Channel]  pinPolCh4=Active Low  pinPolCh5=Active High  outputComplem4=Main duplicated  outputLevel4=High  outputLevel5=Low  pinFtmCh6=PTC12: [FTM3_CH6 | FTM Channel]  pinFtmCh7=None  pinPolCh6=Active Low  pinPolCh7=Active Low  outputComplem6=Main duplicated  outputLevel6=Low  outputLevel7=Low  initTrigger=off  chTrigger0=off  chTrigger1=off  chTrigger2=off  chTrigger3=off  chTrigger4=off  chTrigger5=off  chTrigger6=off  chTrigger7=off  mcuTargetUpdate=on  pwmSyncTrg=Software trigger  pwmSyncHwRouting=TRGMUX_FTM7  pwmSyncTrg0=off  pwmSyncTrg1=off  pwmSyncTrg2=off  pwmSyncAutoClear=off  pwmSyncMinLoad=off  pwmSyncMaxLoad=on  pwmSyncInvert=PWM Syncronization  pwmSyncOutControl=PWM Syncronization  pwmSyncOutMask=PWM Syncronization  pwmSyncCounterInitial=PWM Syncronization  pwmSyncPoints=Wait Loading Points  reloadEnable=off  reloadPriority=15  reloadHalfCycle=off  reloadHCR=0  reloadFrequency=0  chnMatch0=off  chnMatch1=off  chnMatch2=off  chnMatch3=off  chnMatch4=off  chnMatch5=off  chnMatch6=off  chnMatch7=off  pwmFaultProtection=off  pwmFaultInterrupt=off  pwmFaultClearing=Fault control disabled  pwmFaultPinState=Safe Value  pwmFaultFilterValue=0  pwmFaultPriority=15  fault_disen_0=off  fault_filter_0=off  fault_polarity_0=Active High  fault_disen_1=off  fault_filter_1=off  fault_polarity_1=Active high  fault_disen_2=off  fault_filter_2=off  fault_polarity_2=Active high  fault_disen_3=off  fault_filter_3=off  fault_polarity_3=Active high  fault_pin_0=None  fault_pin_1=None  fault_pin_2=None  fault_pin_3=None
  Mux2 : Mux  Inputs=3
  Switch4 : Switch  Threshold=0.5  RndMeth=Simplest
  stop : Constant  Value=0  OutDataTypeStr=single
  wires:
  PWM_Duty Cycle/1 -> Switch4/1
  Mux2/1 -> Switch4/3
  Switch4/1 -> Demux1/1
  stop/1 -> Mux2/1, Mux2/3, Mux2/2
  EnPWM/1 -> Switch4/2
  Demux1/1 -> FTM_PWM_Config/1  "PWM_A"
  Demux1/2 -> FTM_PWM_Config/2  "PWM_B"
  Demux1/3 -> FTM_PWM_Config/3  "PWM_C"

== system mcb_pmsm_hall_offset_MCSPTE1AK144/Offset Calculation/Subsystem1 ==
  Iab_meas_ADC : Inport
  Calculate Position from Hall : Subsystem
  Terminator : Terminator
  Pos_PU : Outport  VectorParamsAs1DForOutWhenUnconnected=off
  wires:
  Iab_meas_ADC/1 -> Terminator/1
  Calculate Position from Hall/1(Pos_PU) -> Pos_PU/1

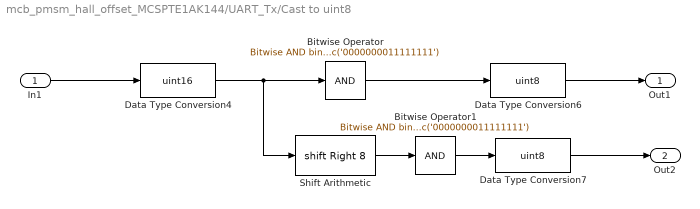
== system mcb_pmsm_hall_offset_MCSPTE1AK144/UART_Tx/Cast to uint8 ==
  In1 : Inport
  Bitwise Operator : simulink/Logic and Bit Operations/Bitwise Operator  logicop=AND  UseBitMask=on  BitMask=bin2dec('0000000011111111')  BitMaskRealWorld=Stored Integer
  Bitwise Operator1 : simulink/Logic and Bit Operations/Bitwise Operator  logicop=AND  UseBitMask=on  BitMask=bin2dec('0000000011111111')  BitMaskRealWorld=Stored Integer
  Data Type Conversion4 : DataTypeConversion  OutDataTypeStr=uint16  ConvertRealWorld=Stored Integer (SI)  RndMeth=Simplest
  Data Type Conversion6 : DataTypeConversion  OutDataTypeStr=uint8  RndMeth=Simplest
  Data Type Conversion7 : DataTypeConversion  OutDataTypeStr=uint8  RndMeth=Simplest
  Shift Arithmetic : ArithShift  BitShiftNumber=8  BitShiftDirection=Right
  Out1 : Outport
  Out2 : Outport  Port=2
  wires:
  Bitwise Operator/1 -> Data Type Conversion6/1
  Data Type Conversion4/1 -> Shift Arithmetic/1, Bitwise Operator/1
  In1/1 -> Data Type Conversion4/1
  Bitwise Operator1/1 -> Data Type Conversion7/1
  Data Type Conversion7/1 -> Out2/1
  Shift Arithmetic/1 -> Bitwise Operator1/1
  Data Type Conversion6/1 -> Out1/1

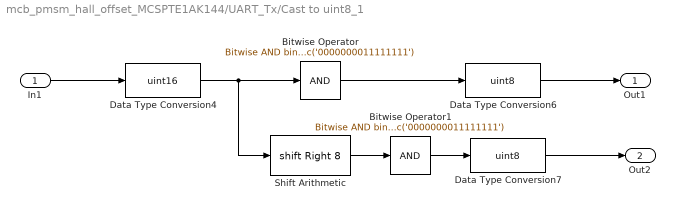
== system mcb_pmsm_hall_offset_MCSPTE1AK144/UART_Tx/Cast to uint8_1 ==
  In1 : Inport
  Bitwise Operator : simulink/Logic and Bit Operations/Bitwise Operator  logicop=AND  UseBitMask=on  BitMask=bin2dec('0000000011111111')  BitMaskRealWorld=Stored Integer
  Bitwise Operator1 : simulink/Logic and Bit Operations/Bitwise Operator  logicop=AND  UseBitMask=on  BitMask=bin2dec('0000000011111111')  BitMaskRealWorld=Stored Integer
  Data Type Conversion4 : DataTypeConversion  OutDataTypeStr=uint16  ConvertRealWorld=Stored Integer (SI)  RndMeth=Simplest
  Data Type Conversion6 : DataTypeConversion  OutDataTypeStr=uint8  RndMeth=Simplest
  Data Type Conversion7 : DataTypeConversion  OutDataTypeStr=uint8  RndMeth=Simplest
  Shift Arithmetic : ArithShift  BitShiftNumber=8  BitShiftDirection=Right
  Out1 : Outport
  Out2 : Outport  Port=2
  wires:
  Data Type Conversion6/1 -> Out1/1
  Shift Arithmetic/1 -> Bitwise Operator1/1
  Data Type Conversion7/1 -> Out2/1
  Bitwise Operator1/1 -> Data Type Conversion7/1
  In1/1 -> Data Type Conversion4/1
  Data Type Conversion4/1 -> Bitwise Operator/1, Shift Arithmetic/1
  Bitwise Operator/1 -> Data Type Conversion6/1

== system mcb_pmsm_hall_offset_MCSPTE1AK144/Hardware Init/enable_FTM_PDB_ADC_triggering/Custom code to reload the PDB value1 ==

== system mcb_pmsm_hall_offset_MCSPTE1AK144/Offset Calculation/Control_System/PosGen ==
  Enable : EnablePort  StatesWhenEnabling=reset  ShowOutputPort=on
  Compare To Constant : simulink/Logic and Bit Operations/Compare To Constant  relop=<=  const=20 * PWM_frequency / 2  OutDataTypeStr=boolean
  Disable host after 22 seconds : simulink/Logic and Bit Operations/Compare To Constant  relop=<=  const=22 * PWM_frequency / 2  OutDataTypeStr=boolean
  Subsystem1 : Subsystem
  Up Counter : Subsystem
  Theta : Outport
  EnPWM : Outport  Port=2  OutputWhenDisabled=reset  InitialOutput=0  VectorParamsAs1DForOutWhenUnconnected=off
  EnableHost : Outport  Port=3  OutputWhenDisabled=reset  InitialOutput=0  VectorParamsAs1DForOutWhenUnconnected=off
  wires:
  Subsystem1/1(Eps) -> Theta/1
  Enable/1 -> Up Counter/Enable
  Compare To Constant/1 -> EnPWM/1
  Disable host after 22 seconds/1 -> EnableHost/1
  Up Counter/1(Count) -> Disable host after 22 seconds/1, Compare To Constant/1, Subsystem1/1(Count)

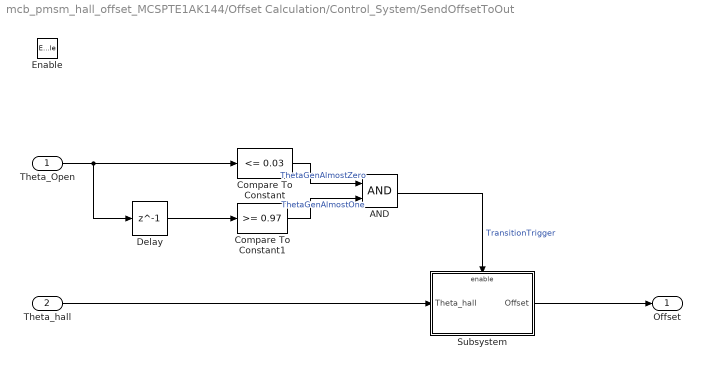
== system mcb_pmsm_hall_offset_MCSPTE1AK144/Offset Calculation/Control_System/SendOffsetToOut ==
  Theta_Open : Inport
  Theta_hall : Inport  Port=2
  Enable : EnablePort  StatesWhenEnabling=reset
  AND : Logic  AllPortsSameDT=off  OutDataTypeStr=boolean
  Compare To Constant : simulink/Logic and Bit Operations/Compare To Constant  relop=<=  const=0.03  OutDataTypeStr=boolean
  Compare To Constant1 : simulink/Logic and Bit Operations/Compare To Constant  relop=>=  const=0.97  OutDataTypeStr=boolean
  Delay : Delay  DelayLength=1
  Subsystem : Subsystem
  Offset : Outport
  wires:
  Theta_Open/1 -> Delay/1, Compare To Constant/1
  Delay/1 -> Compare To Constant1/1
  Compare To Constant/1 -> AND/1  "ThetaGenAlmostZero"
  Compare To Constant1/1 -> AND/2  "ThetaGenAlmostOne"
  Theta_hall/1 -> Subsystem/1(Theta_hall)
  AND/1 -> Subsystem/Enable  "TransitionTrigger"
  Subsystem/1(Offset) -> Offset/1

== system mcb_pmsm_hall_offset_MCSPTE1AK144/Offset Calculation/Control_System/Subsystem1 ==
  Input : Inport
  Enable : EnablePort
  Offset : Outport
  wires:
  Input/1 -> Offset/1

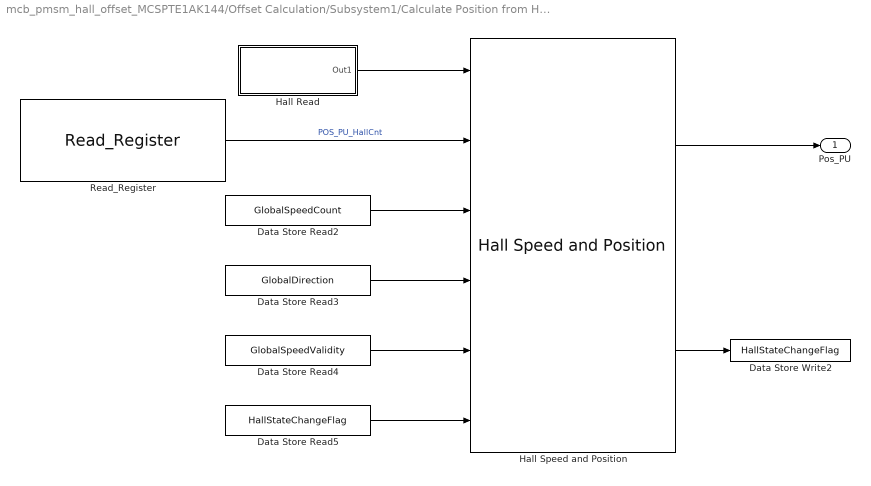
== system mcb_pmsm_hall_offset_MCSPTE1AK144/Offset Calculation/Subsystem1/Calculate Position from Hall ==
  Data Store Read2 : DataStoreRead  DataStoreName=GlobalSpeedCount  IndexOptions=Index vector (dialog)  Indices=1  OutputSizes=1
  Data Store Read3 : DataStoreRead  DataStoreName=GlobalDirection  IndexOptions=Index vector (dialog)  Indices=1  OutputSizes=1
  Data Store Read4 : DataStoreRead  DataStoreName=GlobalSpeedValidity  IndexOptions=Index vector (dialog)  Indices=1  OutputSizes=1
  Data Store Read5 : DataStoreRead  Priority=1  DataStoreName=HallStateChangeFlag  IndexOptions=Index vector (dialog)  Indices=1  OutputSizes=1
  Data Store Write2 : DataStoreWrite  Priority=2  DataStoreName=HallStateChangeFlag  IndexOptions=Index vector (dialog)  Indices=1  OutputSizes=1
  Hall Read : Subsystem
  Hall Speed and Position : mcbpositiondecoderlib/Hall Speed and Position  blkExecutionType=Position  CounterSize=16 bits  ClkFreq=80000000/128  BlkSampleTime=Ts  PolePairs=pmsm.p  MinSpeed=50  HallInterruptConfig=Every 60 Degrees  SpeedUnit=Per unit  PerUnitSpeed=pmsm.N_max  SpeedDataType=dataType  hallSequence=ABC  Sequence=[5,4,6,2,3,1]  EnableSecondOrder=1st Order  PositionUnit=Per unit  PositionDataType=dataType
      settings: SourceProductBaseCode=MT
  Read_Register : mbd_s32k1xx_ec_toolbox/Utility Blocks/Read_Register  periph=ADC0  reg=SC1A  addr=0x4003A004  regSize=32  pcc_clock=ADC0_CLK
  Pos_PU : Outport  InitialOutput=0  VectorParamsAs1DForOutWhenUnconnected=off
  wires:
  Hall Speed and Position/2 -> Data Store Write2/1
  Data Store Read5/1 -> Hall Speed and Position/6
  Data Store Read4/1 -> Hall Speed and Position/5
  Data Store Read2/1 -> Hall Speed and Position/3
  Data Store Read3/1 -> Hall Speed and Position/4
  Hall Speed and Position/1 -> Pos_PU/1
  Read_Register/1 -> Hall Speed and Position/2  "POS_PU_HallCnt"
  Hall Read/1(Out1) -> Hall Speed and Position/1

== system mcb_pmsm_hall_offset_MCSPTE1AK144/Offset Calculation/Control_System/PosGen/Subsystem1 ==
  Count : Inport
  Count for 2.5 sec : Constant  Value=2.5 * PWM_frequency / 2  OutDataTypeStr=uint32  SampleTime=-1
  If : If  NumInputs=2  IfExpression=u1 < u2
  If Action Subsystem : Subsystem  TreatAsAtomicUnit=on
  If Action Subsystem2 : Subsystem  TreatAsAtomicUnit=on
  Merge : Merge
  Position Generator : mcbcontrolslib/Position Generator  AngleOutput=Per-unit  ThetaSource=External  ThetaInput=5e-4  DataType=double  ExternalReset=none  Offset=0
      settings: SourceProductBaseCode=MT
  Eps : Outport
  wires:
  If Action Subsystem/1(Out1) -> Merge/1
  If/1 -> If Action Subsystem/Action
  If Action Subsystem2/1(Out1) -> Merge/2
  Position Generator/1 -> Eps/1
  Count/1 -> If/1
  Merge/1 -> Position Generator/1  "DeltaT"
  If/2 -> If Action Subsystem2/Action
  Count for 2.5 sec/1 -> If/2

== system mcb_pmsm_hall_offset_MCSPTE1AK144/Offset Calculation/Control_System/PosGen/Up Counter ==
  Enable : EnablePort  StatesWhenEnabling=reset
  Add1 : Sum  SaturateOnIntegerOverflow=on
  Constant : Constant  OutDataTypeStr=uint32
  Delay : Delay  DelayLength=1
  Count : Outport  OutputWhenDisabled=reset  InitialOutput=0
  wires:
  Add1/1 -> Count/1, Delay/1
  Constant/1 -> Add1/1
  Delay/1 -> Add1/2

== system mcb_pmsm_hall_offset_MCSPTE1AK144/Offset Calculation/Control_System/SendOffsetToOut/Subsystem ==
  Theta_hall : Inport
  Enable : EnablePort
  IIR Filter : mcbcontrolslib/IIR Filter  VariantControl=Low Pass Filter  VariantSelect=Low-pass  Filter_constant=0.5  advancedSettings=off  Ts=50e-6  cutOff_freq=3183.0989
      settings: SourceProductBaseCode=MT
  Offset : Outport
  wires:
  IIR Filter/1 -> Offset/1
  Theta_hall/1 -> IIR Filter/1

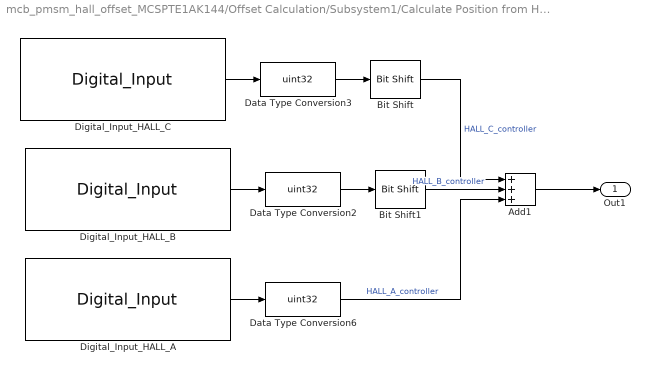
== system mcb_pmsm_hall_offset_MCSPTE1AK144/Offset Calculation/Subsystem1/Calculate Position from Hall/Hall Read ==
  Add1 : Sum  Inputs=+++  OutDataTypeStr=Inherit: Inherit via back propagation
  Bit Shift : hdlsllib/Logic and Bit Operations/Bit Shift  mode=Shift Left Logical  N=2
  Bit Shift1 : hdlsllib/Logic and Bit Operations/Bit Shift  mode=Shift Left Logical  N=1
  Data Type Conversion2 : DataTypeConversion  OutDataTypeStr=uint32
  Data Type Conversion3 : DataTypeConversion  OutDataTypeStr=uint32
  Data Type Conversion6 : DataTypeConversion  OutDataTypeStr=uint32
  Digital_Input_HALL_A : mbd_s32k1xx_ec_toolbox/GPIO Blocks/Digital_Input  gpio_pin=PTD11: [PTD11 | Port D I/O]  pull_resistor=None  passive_filter=off
  Digital_Input_HALL_B : mbd_s32k1xx_ec_toolbox/GPIO Blocks/Digital_Input  gpio_pin=PTD10: [PTD10 | Port D I/O]  pull_resistor=None  passive_filter=off
  Digital_Input_HALL_C : mbd_s32k1xx_ec_toolbox/GPIO Blocks/Digital_Input  gpio_pin=PTA1: [PTA1 | Port A I/O]  pull_resistor=None  passive_filter=off
  Out1 : Outport
  wires:
  Add1/1 -> Out1/1
  Data Type Conversion2/1 -> Bit Shift1/1
  Bit Shift/1 -> Add1/1  "HALL_C_controller"
  Bit Shift1/1 -> Add1/2  "HALL_B_controller"
  Data Type Conversion6/1 -> Add1/3  "HALL_A_controller"
  Data Type Conversion3/1 -> Bit Shift/1
  Digital_Input_HALL_C/1 -> Data Type Conversion3/1
  Digital_Input_HALL_B/1 -> Data Type Conversion2/1
  Digital_Input_HALL_A/1 -> Data Type Conversion6/1

== system mcb_pmsm_hall_offset_MCSPTE1AK144/Offset Calculation/Control_System/PosGen/Subsystem1/If Action Subsystem ==
  Action Port : ActionPort  ActionPortLabel=if(u1 < u2)
  Constant : Constant  Value=0  OutDataTypeStr=dataType
  Out1 : Outport
  wires:
  Constant/1 -> Out1/1

== system mcb_pmsm_hall_offset_MCSPTE1AK144/Offset Calculation/Control_System/PosGen/Subsystem1/If Action Subsystem2 ==
  Action Port : ActionPort  ActionPortLabel=else
  Add1 : Sum
  Constant1 : Constant  Value=1e-3  OutDataTypeStr=dataType
  Delay : Delay  DelayLength=1
  Multiply : Gain  Gain=Ts  OutDataTypeStr=Inherit: Same as input
  Saturation1 : Saturate  UpperLimit=2 * pmsm.p  LowerLimit=0
  Out1 : Outport
  wires:
  Delay/1 -> Add1/2
  Constant1/1 -> Add1/1
  Add1/1 -> Saturation1/1
  Multiply/1 -> Out1/1
  Saturation1/1 -> Delay/1, Multiply/1

== stateflow chart mcb_pmsm_hall_offset_MCSPTE1AK144/Hardware Init/Enable PDB and start FTM ==
  settings: sampleTime=0.500
  state A
  state END
  (default) -> A
  A -> END : {enablePDB;}
  END -> END : {Normal_Op;}
  events: enablePDB output FUNCTION_CALL_EVENT; Normal_Op output FUNCTION_CALL_EVENT
